simulink model "modelStab"  (R2013b)
settings: Solver=ode4  StartTime=0.0  StopTime=tSim  FixedStep=h  RelTol=1e-3
values from neighbouring files (symbols this model uses):
  modelSelect = 'full'    [launcher_script.m]    (also in launcher_simulink.m = 'linear')
  params = [M,m,L,I,b,g]    [launcher_script.m]    (also in launcher_simulink.m)
  state0 = [thetaDot0;theta0;xDot0;x0]    [launcher_script.m]    (also in launcher_simulink.m; sFunction.m = [])
settings Model: Creator=JAR  LastModifiedBy=JAR

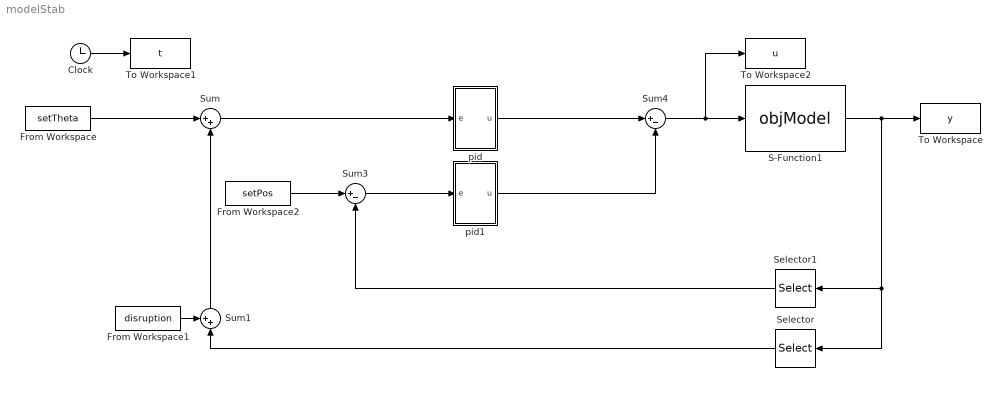
== system modelStab ==
  Clock : Clock
  From Workspace : FromWorkspace  VariableName=setTheta  SampleTime=0
  From Workspace1 : FromWorkspace  VariableName=disruption  SampleTime=0
  From Workspace2 : FromWorkspace  VariableName=setPos  SampleTime=0
  S-Function1 : S-Function  FunctionName=objModel  Parameters=state0,params,modelSelect  EnableBusSupport=off
  Selector : Selector  InputPortWidth=4  IndexOptions=Index vector (dialog)  Indices=2  OutputSizes=1
  Selector1 : Selector  InputPortWidth=4  IndexOptions=Index vector (dialog)  Indices=4  OutputSizes=1
  Sum : Sum  Inputs=|++
  Sum1 : Sum  Inputs=++|
  Sum3 : Sum  Inputs=|+-
  Sum4 : Sum  Inputs=|+-
  To Workspace : ToWorkspace  VariableName=y  SampleTime=-1
  To Workspace1 : ToWorkspace  VariableName=t  SampleTime=-1
  To Workspace2 : ToWorkspace  VariableName=u  SampleTime=-1
  pid : Subsystem
  pid1 : Subsystem
  wires:
  Clock/1 -> To Workspace1/1
  From Workspace1/1 -> Sum1/1
  Sum1/1 -> Sum/2
  S-Function1/1 -> Selector1/1, Selector/1, To Workspace/1
  Selector/1 -> Sum1/2
  From Workspace/1 -> Sum/1
  From Workspace2/1 -> Sum3/1
  Selector1/1 -> Sum3/2
  Sum4/1 -> To Workspace2/1, S-Function1/1
  Sum/1 -> pid/1(e)
  pid/1(u) -> Sum4/1
  Sum3/1 -> pid1/1(e)
  pid1/1(u) -> Sum4/2

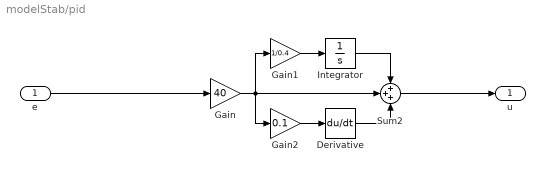
== system modelStab/pid ==
  e : Inport
  Derivative : Derivative
  Gain : Gain  Gain=40
  Gain1 : Gain  Gain=1/0.4
  Gain2 : Gain  Gain=0.1
  Integrator : Integrator
  Sum2 : Sum  Inputs=+++
  u : Outport
  wires:
  Sum2/1 -> u/1
  Gain1/1 -> Integrator/1
  Gain/1 -> Gain2/1, Gain1/1, Sum2/2
  e/1 -> Gain/1
  Derivative/1 -> Sum2/3
  Integrator/1 -> Sum2/1
  Gain2/1 -> Derivative/1

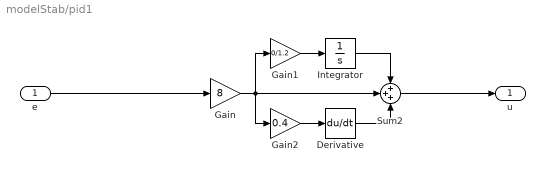
== system modelStab/pid1 ==
  e : Inport
  Derivative : Derivative
  Gain : Gain  Gain=8
  Gain1 : Gain  Gain=0/1.2
  Gain2 : Gain  Gain=0.4
  Integrator : Integrator
  Sum2 : Sum  Inputs=+++
  u : Outport
  wires:
  Sum2/1 -> u/1
  Gain1/1 -> Integrator/1
  Gain/1 -> Gain2/1, Gain1/1, Sum2/2
  e/1 -> Gain/1
  Derivative/1 -> Sum2/3
  Integrator/1 -> Sum2/1
  Gain2/1 -> Derivative/1
